simulink model "Problem_8_Chart"  (R2020a)
settings: Solver=VariableStepAuto  StartTime=0.0  StopTime=10.0  RelTol=1e-3
settings Model: Creator=Admin  LastModifiedBy=Admin

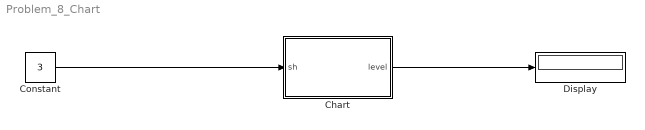
== system Problem_8_Chart ==
  Chart : Stateflow chart  TreatAsAtomicUnit=on
  Constant : Constant  Value=3
  Display : Display
  wires:
  Chart/1(level) -> Display/1
  Constant/1 -> Chart/1(sh)

== stateflow chart Problem_8_Chart/Chart ==
  state Floor_1
    entry:
    cur_st=1;
    level=1;
  state Floor_2
    entry:
    level=2;
    cur_st=level;
  state Floor_3
    entry:
    level=3;
    cur_st=level;
  state Floor_4
    entry:
    level=4;
    cur_st=level;
  state Floor_5
    entry:
    level=5;
    cur_st=level;
  (default) -> Floor_1
  Floor_5 -> Floor_5 [order 2] : [cur_st==5]
  Floor_4 -> Floor_5 [order 1] : [cur_st<sh]
  Floor_3 -> Floor_4 [order 1] : [cur_st<sh]
  Floor_1 -> Floor_2 [order 1] : [cur_st<sh]
  Floor_2 -> Floor_3 [order 1] : [cur_st<sh]
  Floor_1 -> Floor_1 [order 2] : [cur_st==1]
  Floor_4 -> Floor_3 [order 2] : [cur_st>sh]
  Floor_3 -> Floor_2 [order 2] : [cur_st>sh]
  Floor_2 -> Floor_1 [order 2] : [cur_st>sh]
  Floor_5 -> Floor_4 [order 1] : [cur_st>sh]
  data: sh input; cur_st local =0; level output
